simulink model "Aufgabe2_3"  (R2025b)
settings: Solver=ode45  StartTime=0.0  StopTime=10  FixedStep=0.05  RelTol=1e-9
libraries: simulink_extras x7
settings Model: Creator=henri  LastModifiedBy=henri

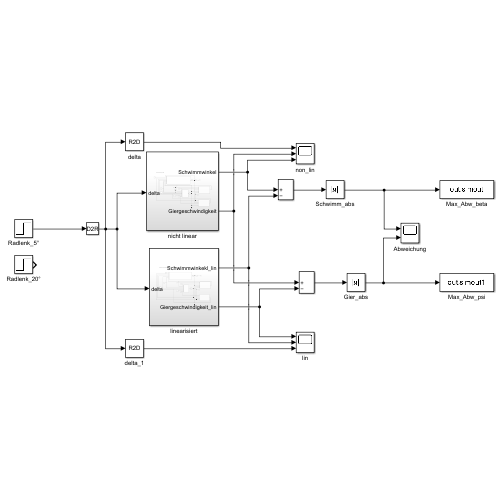
[thumbnail: Simulink's stored preview of the top-level diagram]
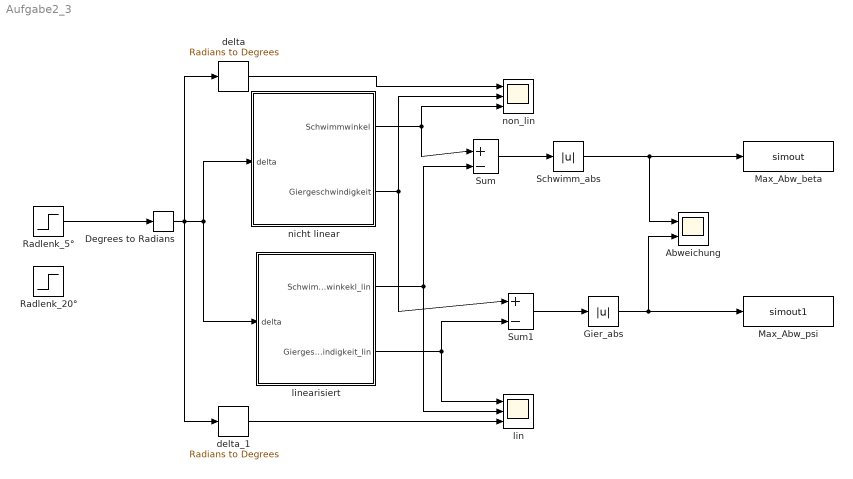
== system Aufgabe2_3 ==
  Abweichung : Scope  NumInputPorts=2
      settings: ActiveDisplayYMinimum=-1  ActiveDisplayYMaximum=1
  Degrees to Radians : simulink_extras/Transformations/Degrees to Radians
  Gier_abs : Abs  SaturateOnIntegerOverflow=off
  Max_Abw_beta : ToWorkspace  VariableName=simout  SaveFormat=Timeseries  SampleTime=-1
  Max_Abw_psi : ToWorkspace  VariableName=simout1  SaveFormat=Timeseries  SampleTime=-1
  Radlenk_20° : Step  After=20  SampleTime=0
  Radlenk_5° : Step  After=5  SampleTime=0
  Schwimm_abs : Abs  SaturateOnIntegerOverflow=off
  Sum : Sum  Inputs=|+-
  Sum1 : Sum  Inputs=|+-
  delta : simulink_extras/Transformations/Radians to Degrees
  delta_1 : simulink_extras/Transformations/Radians to Degrees
  lin : Scope  NumInputPorts=3
      settings: ActiveDisplayYMinimum=-3.28349882771291  ActiveDisplayYMaximum=20.549891365020041  DataLoggingVariableName=ScopeData2
  linearisiert : Subsystem
  nicht linear : Subsystem
  non_lin : Scope  NumInputPorts=3
      settings: ActiveDisplayYMinimum=-3.2734879691070797  ActiveDisplayYMaximum=20.489149584162313
  wires:
  Radlenk_5°/1 -> Degrees to Radians/1
  Degrees to Radians/1 -> delta_1/1, delta/1, linearisiert/1(delta), nicht linear/1(delta)
  linearisiert/1(Schwimmwinkekl_lin) -> Sum/2, lin/2
  nicht linear/1(Schwimmwinkel) -> non_lin/3, Sum/1
  Sum/1 -> Schwimm_abs/1
  linearisiert/2(Giergeschwindigkeit_lin) -> Sum1/2, lin/1
  Sum1/1 -> Gier_abs/1
  nicht linear/2(Giergeschwindigkeit) -> non_lin/2, Sum1/1
  Schwimm_abs/1 -> Abweichung/1, Max_Abw_beta/1
  Gier_abs/1 -> Max_Abw_psi/1, Abweichung/2
  delta_1/1 -> lin/3
  delta/1 -> non_lin/1

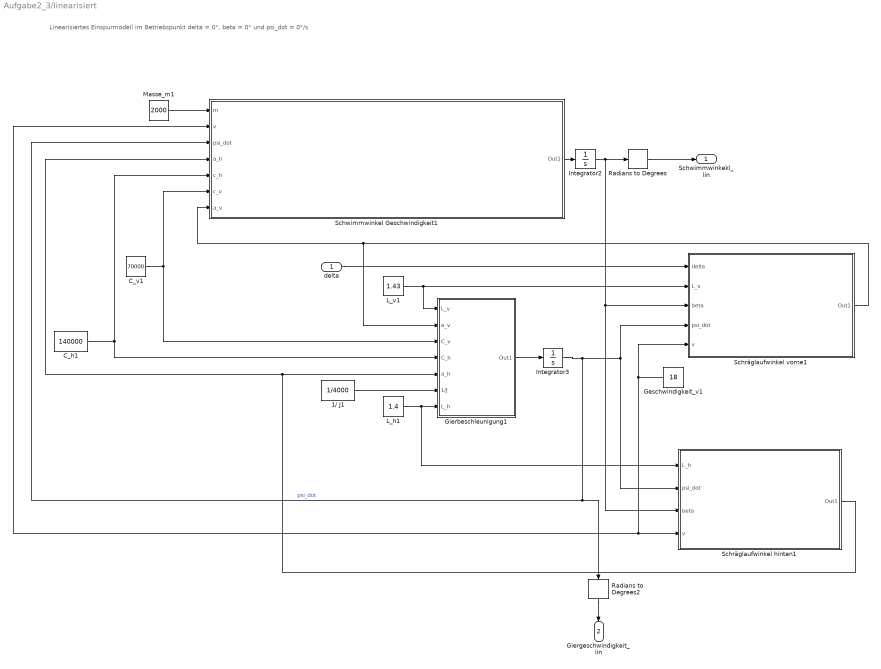
== system Aufgabe2_3/linearisiert ==
  note: Linearisiertes Einspurmodell im Betriebspunkt delta = 0°, beta = 0° und psi_dot = 0°/s
  delta : Inport
  1/ J1 : Constant  Value=1/4000
  C_h1 : Constant  Value=140000
  C_v1 : Constant  Value=70000
  Geschwindigkeit_v1 : Constant  Value=18
  Gierbeschleunigung1 : Subsystem
  Integrator2 : Integrator
  Integrator3 : Integrator
  L_h1 : Constant  Value=1.4
  L_v1 : Constant  Value=1.43
  Masse_m1 : Constant  Value=2000
  Radians to Degrees : simulink_extras/Transformations/Radians to Degrees
  Radians to Degrees2 : simulink_extras/Transformations/Radians to Degrees
  Schräglaufwinkel hinten1 : Subsystem
  Schräglaufwinkel vorne1 : Subsystem
  Schwimmwinkel Geschwindigkeit1 : Subsystem
  Schwimmwinkekl_lin : Outport
  Giergeschwindigkeit_lin : Outport  Port=2
  wires:
  Integrator3/1 -> Schwimmwinkel Geschwindigkeit1/3(psi_dot), Radians to Degrees2/1, Schräglaufwinkel hinten1/2(psi_dot), Schräglaufwinkel vorne1/4(psi_dot)  "psi_dot"
  Schräglaufwinkel hinten1/1(Out1) -> Schwimmwinkel Geschwindigkeit1/4(a_h), Gierbeschleunigung1/5(a_h)
  Integrator2/1 -> Radians to Degrees/1, Schräglaufwinkel vorne1/3(beta), Schräglaufwinkel hinten1/3(beta)
  C_v1/1 -> Schwimmwinkel Geschwindigkeit1/6(c_v), Gierbeschleunigung1/3(C_v)
  Geschwindigkeit_v1/1 -> Schwimmwinkel Geschwindigkeit1/2(v), Schräglaufwinkel hinten1/4(v), Schräglaufwinkel vorne1/5(v)
  L_v1/1 -> Gierbeschleunigung1/1(L_v), Schräglaufwinkel vorne1/2(L_v)
  C_h1/1 -> Gierbeschleunigung1/4(C_h), Schwimmwinkel Geschwindigkeit1/5(c_h)
  Schräglaufwinkel vorne1/1(Out1) -> Gierbeschleunigung1/2(a_v), Schwimmwinkel Geschwindigkeit1/7(a_v)
  Gierbeschleunigung1/1(Out1) -> Integrator3/1
  Schwimmwinkel Geschwindigkeit1/1(Out1) -> Integrator2/1
  1/ J1/1 -> Gierbeschleunigung1/6(1/J)
  L_h1/1 -> Schräglaufwinkel hinten1/1(L_h), Gierbeschleunigung1/7(L_h)
  Masse_m1/1 -> Schwimmwinkel Geschwindigkeit1/1(m)
  delta/1 -> Schräglaufwinkel vorne1/1(delta)
  Radians to Degrees/1 -> Schwimmwinkekl_lin/1
  Radians to Degrees2/1 -> Giergeschwindigkeit_lin/1

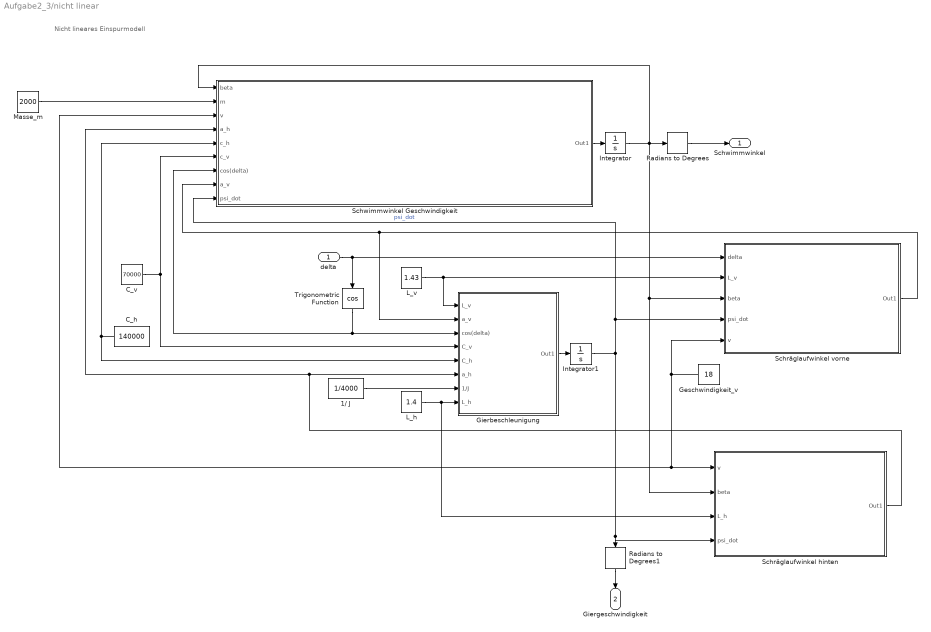
== system Aufgabe2_3/nicht linear ==
  note: Nicht lineares Einspurmodell
  delta : Inport
  1/ J : Constant  Value=1/4000
  C_h : Constant  Value=140000
  C_v : Constant  Value=70000
  Geschwindigkeit_v : Constant  Value=18
  Gierbeschleunigung : Subsystem
  Integrator : Integrator
  Integrator1 : Integrator
  L_h : Constant  Value=1.4
  L_v : Constant  Value=1.43
  Masse_m : Constant  Value=2000
  Radians to Degrees : simulink_extras/Transformations/Radians to Degrees
  Radians to Degrees1 : simulink_extras/Transformations/Radians to Degrees
  Schräglaufwinkel hinten : Subsystem
  Schräglaufwinkel vorne : Subsystem
  Schwimmwinkel Geschwindigkeit : Subsystem
  Trigonometric Function : Trigonometry  Operator=cos
  Schwimmwinkel : Outport
  Giergeschwindigkeit : Outport  Port=2
  wires:
  1/ J/1 -> Gierbeschleunigung/7(1/J)
  Schräglaufwinkel vorne/1(Out1) -> Gierbeschleunigung/2(a_v), Schwimmwinkel Geschwindigkeit/8(a_v)
  Integrator1/1 -> Schräglaufwinkel hinten/4(psi_dot), Radians to Degrees1/1, Schräglaufwinkel vorne/4(psi_dot), Schwimmwinkel Geschwindigkeit/9(psi_dot)  "psi_dot"
  C_v/1 -> Schwimmwinkel Geschwindigkeit/6(c_v), Gierbeschleunigung/4(C_v)
  Geschwindigkeit_v/1 -> Schwimmwinkel Geschwindigkeit/3(v), Schräglaufwinkel hinten/1(v), Schräglaufwinkel vorne/5(v)
  Gierbeschleunigung/1(Out1) -> Integrator1/1
  Integrator/1 -> Schräglaufwinkel vorne/3(beta), Schräglaufwinkel hinten/2(beta), Radians to Degrees/1, Schwimmwinkel Geschwindigkeit/1(beta)
  C_h/1 -> Gierbeschleunigung/5(C_h), Schwimmwinkel Geschwindigkeit/5(c_h)
  L_h/1 -> Schräglaufwinkel hinten/3(L_h), Gierbeschleunigung/8(L_h)
  Schräglaufwinkel hinten/1(Out1) -> Schwimmwinkel Geschwindigkeit/4(a_h), Gierbeschleunigung/6(a_h)
  L_v/1 -> Schräglaufwinkel vorne/2(L_v), Gierbeschleunigung/1(L_v)
  Trigonometric Function/1 -> Gierbeschleunigung/3(cos(delta)), Schwimmwinkel Geschwindigkeit/7(cos(delta))
  Schwimmwinkel Geschwindigkeit/1(Out1) -> Integrator/1
  Masse_m/1 -> Schwimmwinkel Geschwindigkeit/2(m)
  delta/1 -> Schräglaufwinkel vorne/1(delta), Trigonometric Function/1
  Radians to Degrees/1 -> Schwimmwinkel/1
  Radians to Degrees1/1 -> Giergeschwindigkeit/1

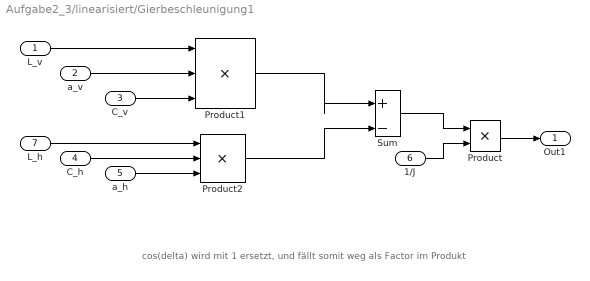
== system Aufgabe2_3/linearisiert/Gierbeschleunigung1 ==
  note: cos(delta) wird mit 1 ersetzt, und fällt somit weg als Factor im Produkt
  L_v : Inport
  a_v : Inport  Port=2
  C_v : Inport  Port=3
  C_h : Inport  Port=4
  a_h : Inport  Port=5
  1/J : Inport  Port=6
  L_h : Inport  Port=7
  Product : Product
  Product1 : Product  Inputs=3
  Product2 : Product  Inputs=3
  Sum : Sum  Inputs=|+-
  Out1 : Outport
  wires:
  Product1/1 -> Sum/1
  Product2/1 -> Sum/2
  a_v/1 -> Product1/2
  1/J/1 -> Product/2
  Sum/1 -> Product/1
  Product/1 -> Out1/1
  a_h/1 -> Product2/3
  C_h/1 -> Product2/2
  L_h/1 -> Product2/1
  L_v/1 -> Product1/1
  C_v/1 -> Product1/3

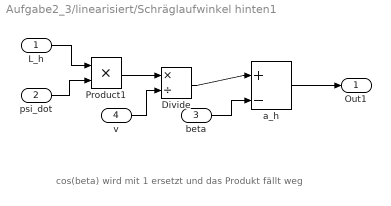
== system Aufgabe2_3/linearisiert/Schräglaufwinkel hinten1 ==
  note: cos(beta) wird mit 1 ersetzt und das Produkt fällt weg
  L_h : Inport
  psi_dot : Inport  Port=2
  beta : Inport  Port=3
  v : Inport  Port=4
  Divide : Product  Inputs=*/
  Product1 : Product
  a_h : Sum  Inputs=|+-
  Out1 : Outport
  wires:
  L_h/1 -> Product1/1
  psi_dot/1 -> Product1/2
  v/1 -> Divide/2
  Product1/1 -> Divide/1
  Divide/1 -> a_h/1
  a_h/1 -> Out1/1
  beta/1 -> a_h/2

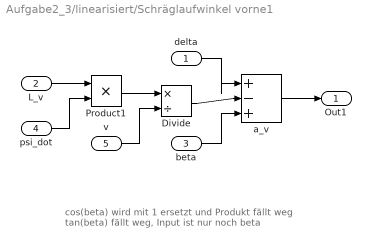
== system Aufgabe2_3/linearisiert/Schräglaufwinkel vorne1 ==
  note: cos(beta) wird mit 1 ersetzt und Produkt fällt weg
      | tan(beta) fällt weg, Input ist nur noch beta
  delta : Inport
  L_v : Inport  Port=2
  beta : Inport  Port=3
  psi_dot : Inport  Port=4
  v : Inport  Port=5
  Divide : Product  Inputs=*/
  Product1 : Product
  a_v : Sum  Inputs=|+-+
  Out1 : Outport
  wires:
  a_v/1 -> Out1/1
  beta/1 -> a_v/3
  Divide/1 -> a_v/2
  delta/1 -> a_v/1
  v/1 -> Divide/2
  Product1/1 -> Divide/1
  psi_dot/1 -> Product1/2
  L_v/1 -> Product1/1

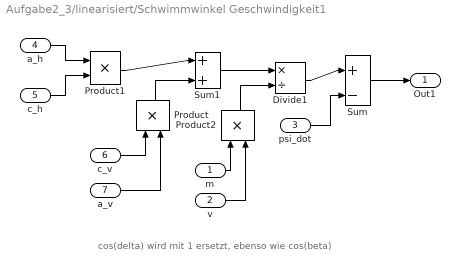
== system Aufgabe2_3/linearisiert/Schwimmwinkel Geschwindigkeit1 ==
  note: cos(delta) wird mit 1 ersetzt, ebenso wie cos(beta)
  m : Inport
  v : Inport  Port=2
  psi_dot : Inport  Port=3
  a_h : Inport  Port=4
  c_h : Inport  Port=5
  c_v : Inport  Port=6
  a_v : Inport  Port=7
  Divide1 : Product  Inputs=*/
  Product : Product
  Product1 : Product
  Product2 : Product
  Sum : Sum  Inputs=|+-
  Sum1 : Sum  Inputs=|++
  Out1 : Outport
  wires:
  c_v/1 -> Product/1
  v/1 -> Product2/2
  c_h/1 -> Product1/2
  Divide1/1 -> Sum/1
  m/1 -> Product2/1
  a_h/1 -> Product1/1
  Product1/1 -> Sum1/1
  psi_dot/1 -> Sum/2
  Product/1 -> Sum1/2
  Product2/1 -> Divide1/2
  Sum1/1 -> Divide1/1
  Sum/1 -> Out1/1
  a_v/1 -> Product/2

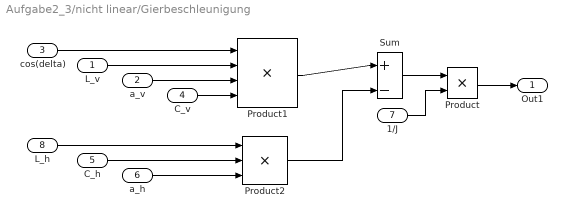
== system Aufgabe2_3/nicht linear/Gierbeschleunigung ==
  L_v : Inport
  a_v : Inport  Port=2
  cos(delta) : Inport  Port=3
  C_v : Inport  Port=4
  C_h : Inport  Port=5
  a_h : Inport  Port=6
  1/J : Inport  Port=7
  L_h : Inport  Port=8
  Product : Product
  Product1 : Product  Inputs=4
  Product2 : Product  Inputs=3
  Sum : Sum  Inputs=|+-
  Out1 : Outport
  wires:
  Product1/1 -> Sum/1
  Product2/1 -> Sum/2
  a_v/1 -> Product1/3
  1/J/1 -> Product/2
  Sum/1 -> Product/1
  cos(delta)/1 -> Product1/1
  Product/1 -> Out1/1
  a_h/1 -> Product2/3
  C_h/1 -> Product2/2
  L_h/1 -> Product2/1
  L_v/1 -> Product1/2
  C_v/1 -> Product1/4

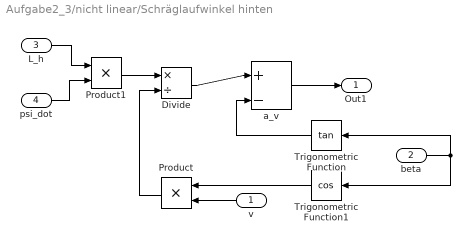
== system Aufgabe2_3/nicht linear/Schräglaufwinkel hinten ==
  v : Inport
  beta : Inport  Port=2
  L_h : Inport  Port=3
  psi_dot : Inport  Port=4
  Divide : Product  Inputs=*/
  Product : Product
  Product1 : Product
  Trigonometric Function : Trigonometry  Operator=tan
  Trigonometric Function1 : Trigonometry  Operator=cos
  a_v : Sum  Inputs=|+-
  Out1 : Outport
  wires:
  L_h/1 -> Product1/1
  v/1 -> Product/2
  beta/1 -> Trigonometric Function1/1, Trigonometric Function/1
  psi_dot/1 -> Product1/2
  Trigonometric Function1/1 -> Product/1
  Product/1 -> Divide/2
  Product1/1 -> Divide/1
  Divide/1 -> a_v/1
  a_v/1 -> Out1/1
  Trigonometric Function/1 -> a_v/2

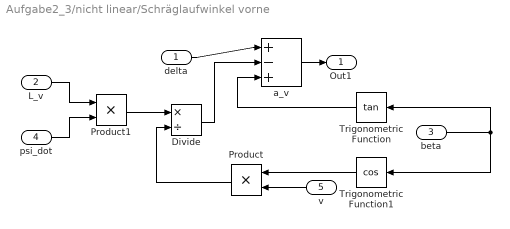
== system Aufgabe2_3/nicht linear/Schräglaufwinkel vorne ==
  delta : Inport
  L_v : Inport  Port=2
  beta : Inport  Port=3
  psi_dot : Inport  Port=4
  v : Inport  Port=5
  Divide : Product  Inputs=*/
  Product : Product
  Product1 : Product
  Trigonometric Function : Trigonometry  Operator=tan
  Trigonometric Function1 : Trigonometry  Operator=cos
  a_v : Sum  Inputs=|+-+
  Out1 : Outport
  wires:
  Product/1 -> Divide/2
  Divide/1 -> a_v/2
  Trigonometric Function1/1 -> Product/1
  L_v/1 -> Product1/1
  v/1 -> Product/2
  Product1/1 -> Divide/1
  Trigonometric Function/1 -> a_v/3
  beta/1 -> Trigonometric Function1/1, Trigonometric Function/1
  delta/1 -> a_v/1
  a_v/1 -> Out1/1
  psi_dot/1 -> Product1/2

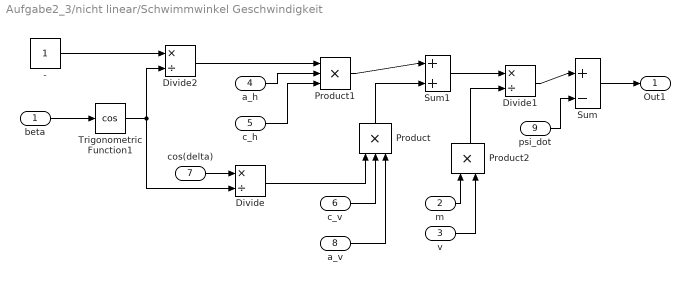
== system Aufgabe2_3/nicht linear/Schwimmwinkel Geschwindigkeit ==
  beta : Inport
  m : Inport  Port=2
  v : Inport  Port=3
  a_h : Inport  Port=4
  c_h : Inport  Port=5
  c_v : Inport  Port=6
  cos(delta) : Inport  Port=7
  a_v : Inport  Port=8
  psi_dot : Inport  Port=9
  - : Constant
  Divide : Product  Inputs=*/
  Divide1 : Product  Inputs=*/
  Divide2 : Product  Inputs=*/
  Product : Product  Inputs=3
  Product1 : Product  Inputs=3
  Product2 : Product
  Sum : Sum  Inputs=|+-
  Sum1 : Sum  Inputs=|++
  Trigonometric Function1 : Trigonometry  Operator=cos
  Out1 : Outport
  wires:
  cos(delta)/1 -> Divide/1
  Divide/1 -> Product/1
  c_v/1 -> Product/2
  v/1 -> Product2/2
  beta/1 -> Trigonometric Function1/1
  c_h/1 -> Product1/3
  Divide1/1 -> Sum/1
  m/1 -> Product2/1
  -/1 -> Divide2/1
  a_h/1 -> Product1/2
  Divide2/1 -> Product1/1
  Product1/1 -> Sum1/1
  Trigonometric Function1/1 -> Divide/2, Divide2/2
  psi_dot/1 -> Sum/2
  a_v/1 -> Product/3
  Product/1 -> Sum1/2
  Product2/1 -> Divide1/2
  Sum1/1 -> Divide1/1
  Sum/1 -> Out1/1
